simulink model "encoderProgramTakeTwo"  (R2019b)
settings: Solver=FixedStepAuto  StartTime=0.0  StopTime=10.0  RelTol=1e-3
libraries: vexarmcortexlib x19, vexcommonlib x3
settings Model: EnablePacing=on  PacingRate=0.100000  ExtModeTrigDuration=25  Creator=jakew  LastModifiedBy=jakew
settings OptimizationCC: EnhancedBackFolding=on  PassReuseOutputArgsAs=Individual arguments  ZeroExternalMemoryAtStartup=off  ZeroInternalMemoryAtStartup=off  MaxStackSize=64  OptimizeBlockOrder=speed  DifferentSizesBufferReuse=on  OptimizationCustomize=off  EfficientTunableParamExpr=on
settings DebuggingCC: ParameterTunabilityLossMsg=error
settings HardwareCC: ProdBitPerPointer=32  ProdBitPerSizeT=32  ProdBitPerPtrDiffT=32  ProdLargestAtomicInteger=Long  ProdLargestAtomicFloat=Double  ProdWordSize=32  ProdHWDeviceType=ARM Compatible->ARM Cortex
settings SFSimCC: MATLABDynamicMemAlloc=off
settings RTWCC: SystemTargetFile=ert.tlc  HardwareBoard=ARM Cortex-based VEX Microcontroller  TLCOptions="-aInlineSetEventsForThisBaseRateFcn=TLC_FALSE -aSuppressMultiTaskScheduler=TLC_FALSE  -aRateBasedStepFcn=0"  TemplateMakefile=ert_default_tmf  GenerateReport=on  Toolchain=GNU Tools for VEX ARM Cortex  IncludeHyperlinkInReport=on  LaunchReport=on  GenerateTraceInfo=on  GenerateTraceReport=on  GenerateTraceReportSl=on  GenerateTraceReportSf=on  GenerateTraceReportEml=on
settings CodeAppCC: ForceParamTrailComments=on  IgnoreCustomStorageClasses=off  OperatorAnnotations=on  SimulinkDataObjDesc=on  SFDataObjDesc=on  InsertBlockDesc=on

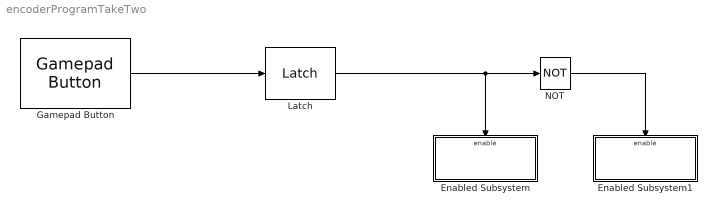
== system encoderProgramTakeTwo ==
  Enabled Subsystem : Subsystem  TreatAsAtomicUnit=on
  Enabled Subsystem1 : Subsystem  TreatAsAtomicUnit=on
  Gamepad Button : vexarmcortexlib/Gamepad/Gamepad Button  joystick=1  chan=7  button56=Up  button78=Up  SimulationIn=off  SampleTime=0.02
      settings: SourceProductName=Simulink Coder Support Package for ARM Cortex-based VEX Microcontroller  SourceProductBaseCode=EC_VEX_MICRO
  Latch : vexcommonlib/Latch  output0=off  BlockPlatform=vexarmcortex
      settings: SourceProductName=Simulink Coder Support Package for ARM Cortex-based VEX Microcontroller  SourceProductBaseCode=EC_VEX_MICRO
  NOT : Logic  Operator=NOT  IconShape=distinctive  AllPortsSameDT=off  OutDataTypeStr=boolean
  wires:
  Latch/1 -> NOT/1, Enabled Subsystem/Enable
  NOT/1 -> Enabled Subsystem1/Enable
  Gamepad Button/1 -> Latch/1

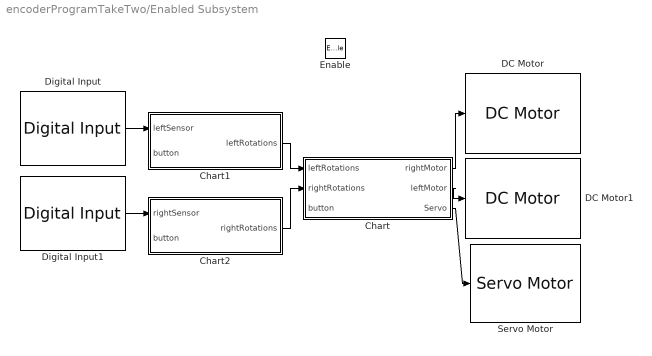
== system encoderProgramTakeTwo/Enabled Subsystem ==
  Enable : EnablePort
  Chart : Stateflow chart  BlockKeywords=__PRM__SERIALIZED__DATA__:Stateflow Chart,Stateflow Diagram  TreatAsAtomicUnit=on
  Chart1 : Stateflow chart  BlockKeywords=__PRM__SERIALIZED__DATA__:Stateflow Chart,Stateflow Diagram  TreatAsAtomicUnit=on
  Chart2 : Stateflow chart  BlockKeywords=__PRM__SERIALIZED__DATA__:Stateflow Chart,Stateflow Diagram  TreatAsAtomicUnit=on
  DC Motor : vexarmcortexlib/Actuators/DC Motor  motor=2  scaleFactor=1/13.5  SimulationOut=off
      settings: SourceProductName=Simulink Coder Support Package for ARM Cortex-based VEX Microcontroller  SourceProductBaseCode=EC_VEX_MICRO
  DC Motor1 : vexarmcortexlib/Actuators/DC Motor  motor=3  scaleFactor=1/13.5  SimulationOut=off
      settings: SourceProductName=Simulink Coder Support Package for ARM Cortex-based VEX Microcontroller  SourceProductBaseCode=EC_VEX_MICRO
  Digital Input : vexarmcortexlib/Sensors/Digital Input  inChan=1  SimulationIn=off  SampleTime=.05
      settings: SourceProductName=Simulink Coder Support Package for ARM Cortex-based VEX Microcontroller  SourceProductBaseCode=EC_VEX_MICRO
  Digital Input1 : vexarmcortexlib/Sensors/Digital Input  inChan=2  SimulationIn=off  SampleTime=.05
      settings: SourceProductName=Simulink Coder Support Package for ARM Cortex-based VEX Microcontroller  SourceProductBaseCode=EC_VEX_MICRO
  Servo Motor : vexarmcortexlib/Actuators/Servo Motor  motor=9  scaleFactor=60/127  SimulationOut=off
      settings: SourceProductName=Simulink Coder Support Package for ARM Cortex-based VEX Microcontroller  SourceProductBaseCode=EC_VEX_MICRO
  wires:
  Chart1/1(leftRotations) -> Chart/1(leftRotations)
  Chart/2(leftMotor) -> DC Motor1/1
  Chart/1(rightMotor) -> DC Motor/1
  Digital Input1/1 -> Chart2/1(rightSensor)
  Chart2/1(rightRotations) -> Chart/2(rightRotations)
  Digital Input/1 -> Chart1/1(leftSensor)
  Chart/3(Servo) -> Servo Motor/1

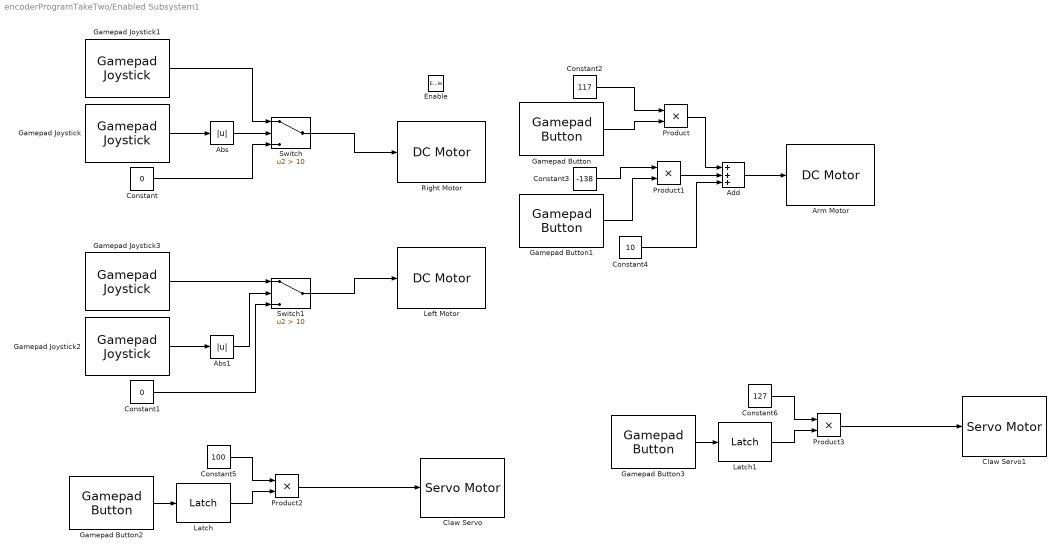
== system encoderProgramTakeTwo/Enabled Subsystem1 ==
  Enable : EnablePort
  Abs : Abs
  Abs1 : Abs
  Add : Sum  Inputs=+++
  "Arm Motor " : vexarmcortexlib/Actuators/DC Motor  motor=8  scaleFactor=1/13.5  SimulationOut=off
      settings: SourceProductName=Simulink Coder Support Package for ARM Cortex-based VEX Microcontroller  SourceProductBaseCode=EC_VEX_MICRO
  Claw Servo : vexarmcortexlib/Actuators/Servo Motor  motor=9  scaleFactor=60/127  SimulationOut=off
      settings: SourceProductName=Simulink Coder Support Package for ARM Cortex-based VEX Microcontroller  SourceProductBaseCode=EC_VEX_MICRO
  Claw Servo1 : vexarmcortexlib/Actuators/Servo Motor  motor=6  scaleFactor=60/127  SimulationOut=off
      settings: SourceProductName=Simulink Coder Support Package for ARM Cortex-based VEX Microcontroller  SourceProductBaseCode=EC_VEX_MICRO
  Constant : Constant  Value=0
  Constant1 : Constant  Value=0
  Constant2 : Constant  Value=117
  Constant3 : Constant  Value=-138
  Constant4 : Constant  Value=10
  Constant5 : Constant  Value=100
  Constant6 : Constant  Value=127
  Gamepad Button : vexarmcortexlib/Gamepad/Gamepad Button  joystick=1  chan=6  button56=Up  button78=Down  SimulationIn=off  SampleTime=0.02
      settings: SourceProductName=Simulink Coder Support Package for ARM Cortex-based VEX Microcontroller  SourceProductBaseCode=EC_VEX_MICRO
  Gamepad Button1 : vexarmcortexlib/Gamepad/Gamepad Button  joystick=1  chan=6  button56=Down  button78=Down  SimulationIn=off  SampleTime=0.02
      settings: SourceProductName=Simulink Coder Support Package for ARM Cortex-based VEX Microcontroller  SourceProductBaseCode=EC_VEX_MICRO
  Gamepad Button2 : vexarmcortexlib/Gamepad/Gamepad Button  joystick=1  chan=5  button56=Up  button78=Down  SimulationIn=off  SampleTime=0.02
      settings: SourceProductName=Simulink Coder Support Package for ARM Cortex-based VEX Microcontroller  SourceProductBaseCode=EC_VEX_MICRO
  Gamepad Button3 : vexarmcortexlib/Gamepad/Gamepad Button  joystick=1  chan=8  button56=Up  button78=Up  SimulationIn=off  SampleTime=0.02
      settings: SourceProductName=Simulink Coder Support Package for ARM Cortex-based VEX Microcontroller  SourceProductBaseCode=EC_VEX_MICRO
  Gamepad Joystick : vexarmcortexlib/Gamepad/Gamepad Joystick  joystick=1  chan=2  SimulationIn=off  SampleTime=0.02
      settings: SourceProductName=Simulink Coder Support Package for ARM Cortex-based VEX Microcontroller  SourceProductBaseCode=EC_VEX_MICRO
  Gamepad Joystick1 : vexarmcortexlib/Gamepad/Gamepad Joystick  joystick=1  chan=2  SimulationIn=off  SampleTime=0.02
      settings: SourceProductName=Simulink Coder Support Package for ARM Cortex-based VEX Microcontroller  SourceProductBaseCode=EC_VEX_MICRO
  Gamepad Joystick2 : vexarmcortexlib/Gamepad/Gamepad Joystick  joystick=1  chan=3  SimulationIn=off  SampleTime=0.02
      settings: SourceProductName=Simulink Coder Support Package for ARM Cortex-based VEX Microcontroller  SourceProductBaseCode=EC_VEX_MICRO
  Gamepad Joystick3 : vexarmcortexlib/Gamepad/Gamepad Joystick  joystick=1  chan=3  SimulationIn=off  SampleTime=0.02
      settings: SourceProductName=Simulink Coder Support Package for ARM Cortex-based VEX Microcontroller  SourceProductBaseCode=EC_VEX_MICRO
  Latch : vexcommonlib/Latch  output0=off  BlockPlatform=vexarmcortex
      settings: SourceProductName=Simulink Coder Support Package for ARM Cortex-based VEX Microcontroller  SourceProductBaseCode=EC_VEX_MICRO
  Latch1 : vexcommonlib/Latch  output0=off  BlockPlatform=vexarmcortex
      settings: SourceProductName=Simulink Coder Support Package for ARM Cortex-based VEX Microcontroller  SourceProductBaseCode=EC_VEX_MICRO
  Left Motor : vexarmcortexlib/Actuators/DC Motor  motor=3  scaleFactor=1/13.5  SimulationOut=off
      settings: SourceProductName=Simulink Coder Support Package for ARM Cortex-based VEX Microcontroller  SourceProductBaseCode=EC_VEX_MICRO
  Product{,1..3} (4 alike) : Product
  Right Motor : vexarmcortexlib/Actuators/DC Motor  motor=2  scaleFactor=1/13.5  SimulationOut=off
      settings: SourceProductName=Simulink Coder Support Package for ARM Cortex-based VEX Microcontroller  SourceProductBaseCode=EC_VEX_MICRO
  Switch : Switch  Criteria=u2 > Threshold  Threshold=10
  Switch1 : Switch  Criteria=u2 > Threshold  Threshold=10
  wires:
  Constant5/1 -> Product2/1
  Gamepad Joystick3/1 -> Switch1/1
  Constant2/1 -> Product/1
  Latch1/1 -> Product3/2
  Switch/1 -> Right Motor/1
  Abs/1 -> Switch/2
  Product3/1 -> Claw Servo1/1
  Latch/1 -> Product2/2
  Constant4/1 -> Add/3
  Gamepad Button1/1 -> Product1/2
  Constant6/1 -> Product3/1
  Gamepad Button2/1 -> Latch/1
  Constant1/1 -> Switch1/3
  Gamepad Joystick1/1 -> Switch/1
  Product2/1 -> Claw Servo/1
  Constant3/1 -> Product1/1
  Add/1 -> "Arm Motor "/1
  Gamepad Button3/1 -> Latch1/1
  Switch1/1 -> Left Motor/1
  Product/1 -> Add/1
  Gamepad Joystick/1 -> Abs/1
  Gamepad Button/1 -> Product/2
  Abs1/1 -> Switch1/2
  Product1/1 -> Add/2
  Gamepad Joystick2/1 -> Abs1/1
  Constant/1 -> Switch/3

== stateflow chart encoderProgramTakeTwo/Enabled Subsystem/Chart ==
  state Straight
    leftMotor = 100;
    rightMotor = 100;
    Servo = 127;
  state CloseClaw
    leftMotor = 0;
    rightMotor= 0;
    Servo = 127;
  state Right
    rightMotor = 100;
    leftMotor = 0;
    Servo = 127;
  state Left
    rightMotor = 0;
    leftMotor = 100;
    Servo = 127;
  state BackUp
    leftMotor = -100;
    rightMotor = -100;
  state Release
    leftMotor = 0;
    rightMotor = 0;
    Servo = 0;
  state Stop
    leftMotor = 0;
    rightMotor = 0;
    Servo = 127;
  CloseClaw -> Straight : after(5,sec)
  (default) -> Straight
  Straight -> Right [order 3] : [leftRotations > (rightRotations)]
  Straight -> Left [order 2] : [rightRotations > (leftRotations)]
  Right -> Straight [order 3] : [rightRotations == leftRotations]
  Left -> Straight [order 2] : [rightRotations == leftRotations]
  Straight -> Stop [order 1] : [rightRotations >= 29 || leftRotations >= 29]
  Stop -> Straight [order 1] : [rightRotations<29 && leftRotations<29]
  BackUp -> CloseClaw : after(.5,sec)
  Right -> Left [order 1] : [rightRotations > (leftRotations)]
  Release -> BackUp : after(.5, sec)
  Left -> Right [order 3] : [leftRotations > (rightRotations)]
  Right -> Stop [order 2] : [rightRotations >= 29 || leftRotations >= 29]
  Left -> Stop [order 1] : [rightRotations >= 29 || leftRotations >=29]
  Stop -> Release [order 2] : after(2,sec)
  data: leftRotations input; rightRotations input; rightMotor output; leftMotor output; button input; Servo output

== stateflow chart encoderProgramTakeTwo/Enabled Subsystem/Chart1 ==
  state OverBlack
    leftRotations = leftRotations + 1;
    leftFlag = 1;
  state Start
    leftRotations = 0;
  state Pause
    leftRotations;
  state Stop
  state OverWhite
    leftRotations = leftRotations + 1;
    leftFlag = 0;
  Start -> OverBlack [order 1] : [leftSensor == 0]
  (default) -> Start
  OverBlack -> Pause
  Pause -> OverBlack [order 2] : [(leftSensor == 0) && (leftFlag == 0)]
  Pause -> OverWhite [order 3] : [(leftSensor == 1) && (leftFlag == 1)]
  Pause -> Stop [order 1] : [leftRotations >= 29]
  OverWhite -> Pause
  Stop -> Start : after(5,sec)
  Start -> OverWhite [order 2] : [leftSensor == 1]
  data: leftSensor input; leftFlag local; leftRotations output; button input

== stateflow chart encoderProgramTakeTwo/Enabled Subsystem/Chart2 ==
  state OverBlack
    rightRotations = rightRotations + 1;
    rightFlag = 1;
  state Start
    rightRotations = 0;
  state Pause
    rightRotations;
  state Stop
  state OverWhite
    rightRotations = rightRotations + 1;
    rightFlag = 0;
  Start -> OverBlack [order 1] : [rightSensor == 0]
  Pause -> OverBlack [order 2] : [(rightSensor == 0) && (rightFlag == 0)]
  (default) -> Start
  OverBlack -> Pause
  Pause -> OverWhite [order 3] : [(rightSensor == 1) && (rightFlag == 1)]
  Pause -> Stop [order 1] : [rightRotations >= 29]
  OverWhite -> Pause
  Stop -> Start : after(5,sec)
  Start -> OverWhite [order 2] : [rightSensor == 1]
  data: rightSensor input; rightRotations output; rightFlag local; button input
